simulink model "penduloInvNoLineal"  (Simulink 7.3)
settings: Solver=ode45  StartTime=0.0  StopTime=0.5  RelTol=1e-3
values from neighbouring files (symbols this model uses):
  K = lqr(A,B,Q,R)    [LQR.m]    (also in bestQ.m = setK_lqr(Q_i); graficosPenduloReal.m = setK_lqr(Q_optimo))
libraries: simulink x5
settings Model: Creator=root  LastModifiedBy=Daniel
settings DebuggingCC: FcnCallInpInsideContextMsg=Enable All  StrictBusMsg=ErrorLevel1
settings GRTTargetCC: CombineOutputUpdateFcns=on

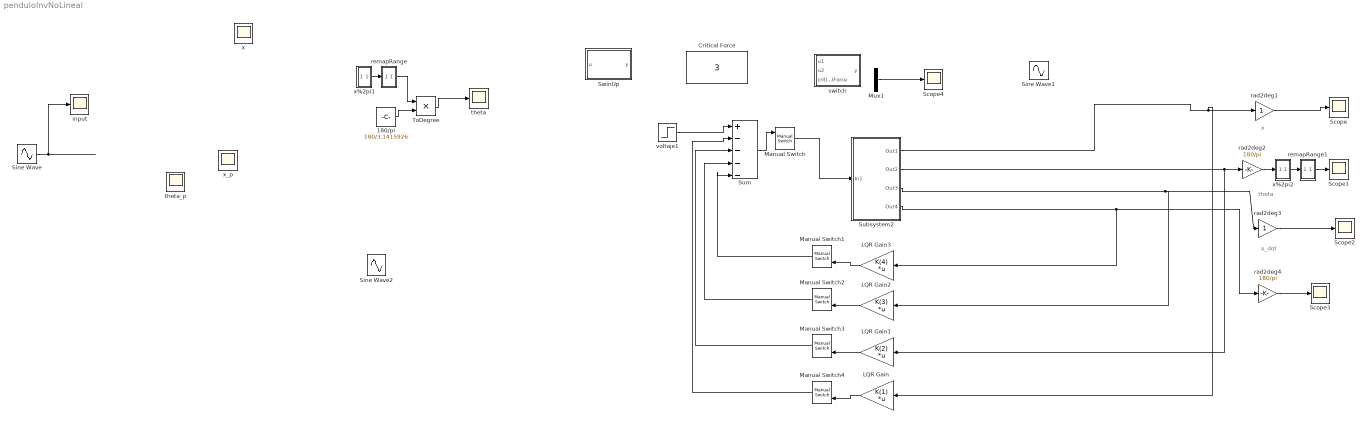
== system penduloInvNoLineal ==
  note: x
  note: theta
  note: x_dot
  180/pi : Constant  Value=180/3.1415926
  Critical Force : Constant  Value=3  OutDataType=fixdt(1, 16)  OutScaling=2^0
  LQR Gain : Gain  Gain=K(1)  Multiplication=Matrix(K*u)  SaturateOnIntegerOverflow=on  OutDataTypeStr=Inherit: Same as input  ParamDataTypeStr=Inherit: Same as input
  LQR Gain1 : Gain  Gain=K(2)  Multiplication=Matrix(K*u)  SaturateOnIntegerOverflow=on  OutDataTypeStr=Inherit: Same as input  ParamDataTypeStr=Inherit: Same as input
  LQR Gain2 : Gain  Gain=K(3)  Multiplication=Matrix(K*u)  SaturateOnIntegerOverflow=on  OutDataTypeStr=Inherit: Same as input  ParamDataTypeStr=Inherit: Same as input
  LQR Gain3 : Gain  Gain=K(4)  Multiplication=Matrix(K*u)  SaturateOnIntegerOverflow=on  OutDataTypeStr=Inherit: Same as input  ParamDataTypeStr=Inherit: Same as input
  Manual Switch : simulink/Signal Routing/Manual Switch  SystemSampleTime=-1  sw=1  action=0  varsize=off
  Manual Switch{1..4} (4 alike) : simulink/Signal Routing/Manual Switch  SystemSampleTime=-1  sw=0  action=0  varsize=off
  Mux1 : Mux  Inputs=2
  Scope{,1..4} (5 alike) : Scope
      Scope settings: SaveName=ScopeData6
      Scope1 settings: SaveName=ScopeData7
      Scope2 settings: SaveName=ScopeData8
      Scope3 settings: SaveName=ScopeData9
      Scope4 settings: SaveName=ScopeData10
  Sine Wave : Sin  Amplitude=0  Bias=0  Frequency=0.25  Phase=0  Samples=10  SampleTime=0.03  Offset=0
  Sine Wave1 : Sin  Amplitude=5  Bias=0  Frequency=1  Phase=0  Samples=10  SampleTime=0  Offset=0
  Sine Wave2 : Sin  Amplitude=2  Bias=0  Frequency=10  Phase=0  Samples=10  SampleTime=0  Offset=0
  Subsystem2 : Subsystem
  Sum : Sum  Inputs=|+----  OutDataType=fixdt(1, 16)  OutScaling=2^0
  SwinUp : Stateflow chart
  ToDegree : Product  RndMeth=Zero
  input : Scope
      settings: SaveName=ScopeData4
  rad2deg1 : Gain  SaturateOnIntegerOverflow=on  OutDataTypeStr=Inherit: Same as input  ParamDataTypeStr=Inherit: Same as input
  rad2deg2 : Gain  Gain=180/pi  SaturateOnIntegerOverflow=on  OutDataTypeStr=Inherit: Same as input  ParamDataTypeStr=Inherit: Same as input
  rad2deg3 : Gain  SaturateOnIntegerOverflow=on  OutDataTypeStr=Inherit: Same as input  ParamDataTypeStr=Inherit: Same as input
  rad2deg4 : Gain  Gain=180/pi  SaturateOnIntegerOverflow=on  OutDataTypeStr=Inherit: Same as input  ParamDataTypeStr=Inherit: Same as input
  remapRange : Stateflow chart  TreatAsAtomicUnit=on
  remapRange1 : Stateflow chart  TreatAsAtomicUnit=on
  switch : Stateflow chart
  theta : Scope
      settings: TimeRange=500  YMin=-200  YMax=200  SaveName=theta
  theta_p : Scope
      settings: SaveName=ScopeData3
  voltaje1 : Step  Time=0  After=1000  SampleTime=0
  x : Scope
  x%2pi1 : Stateflow chart  TreatAsAtomicUnit=on
  x%2pi2 : Stateflow chart  TreatAsAtomicUnit=on
  x_p : Scope
      settings: SaveName=ScopeData2
  wires:
  180/pi/1 -> ToDegree/2
  ToDegree/1 -> theta/1
  x%2pi1/1(y) -> remapRange/1(value)
  remapRange/1(y) -> ToDegree/1
  Sine Wave/1 -> input/1
  ? -> x/1
  ? -> x%2pi1/1(u)
  ? -> x_p/1
  ? -> theta_p/1
  rad2deg4/1 -> Scope3/1
  rad2deg3/1 -> Scope2/1
  Subsystem2/3(Out3) -> LQR Gain2/1, rad2deg3/1
  rad2deg1/1 -> Scope/1
  Mux1/1 -> Scope4/1
  Subsystem2/1(Out1) -> rad2deg1/1, LQR Gain/1
  Subsystem2/2(Out2) -> rad2deg2/1, LQR Gain1/1
  x%2pi2/1(y) -> remapRange1/1(value)
  rad2deg2/1 -> x%2pi2/1(u)
  remapRange1/1(y) -> Scope1/1
  LQR Gain3/1 -> Manual Switch1/2
  LQR Gain2/1 -> Manual Switch2/2
  LQR Gain1/1 -> Manual Switch3/2
  LQR Gain/1 -> Manual Switch4/2
  Manual Switch/1 -> Subsystem2/1(In1)
  Subsystem2/4(Out4) -> rad2deg4/1, LQR Gain3/1
  voltaje1/1 -> Sum/1
  Sum/1 -> Manual Switch/1
  Manual Switch1/1 -> Sum/5
  Manual Switch2/1 -> Sum/4
  Manual Switch3/1 -> Sum/3
  Manual Switch4/1 -> Sum/2

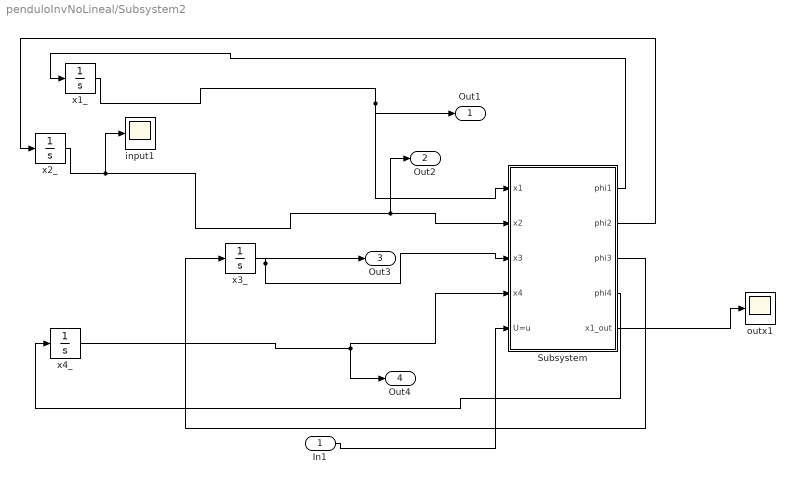
== system penduloInvNoLineal/Subsystem2 ==
  In1 : Inport
  Subsystem : Subsystem
  input1 : Scope
      settings: SaveName=ScopeData5
  outx1 : Scope
  x1_ : Integrator  UpperSaturationLimit=50  LowerSaturationLimit=-50
  x2_ : Integrator  InitialCondition=180.005*pi/180  UpperSaturationLimit=2*pi  LowerSaturationLimit=0
  x3_ : Integrator  UpperSaturationLimit=100  LowerSaturationLimit=-100
  x4_ : Integrator  UpperSaturationLimit=100  LowerSaturationLimit=-100
  Out1 : Outport
  Out2 : Outport  Port=2
  Out3 : Outport  Port=3
  Out4 : Outport  Port=4
  wires:
  x1_/1 -> Subsystem/1(x1), Out1/1
  Subsystem/1(phi1) -> x1_/1
  Subsystem/2(phi2) -> x2_/1
  Subsystem/3(phi3) -> x3_/1
  Subsystem/4(phi4) -> x4_/1
  x4_/1 -> Subsystem/4(x4), Out4/1
  x2_/1 -> input1/1, Subsystem/2(x2), Out2/1
  Subsystem/5(x1_out) -> outx1/1
  In1/1 -> Subsystem/5(U=u)
  x3_/1 -> Out3/1, Subsystem/3(x3)

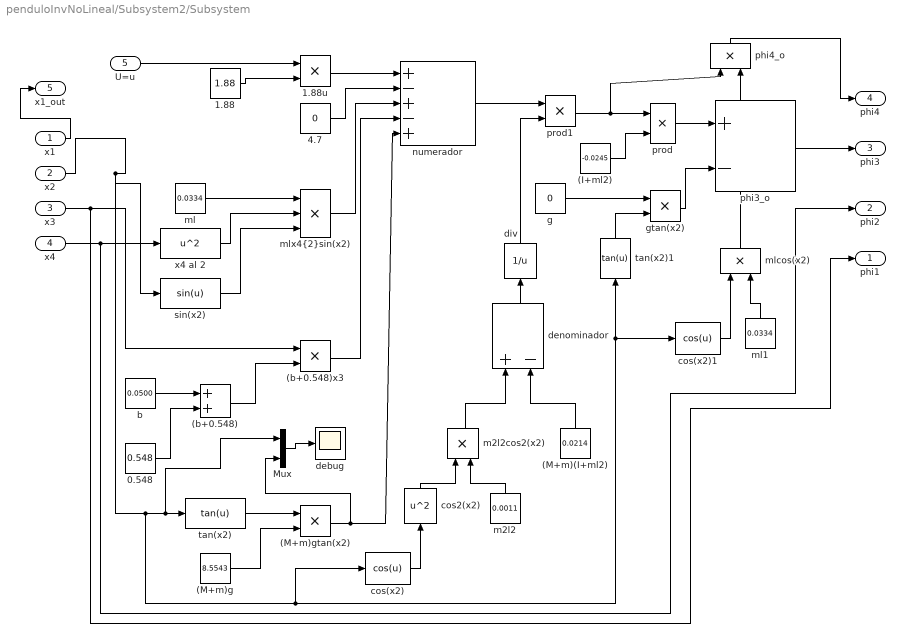
== system penduloInvNoLineal/Subsystem2/Subsystem ==
  x1 : Inport
  x2 : Inport  Port=2
  x3 : Inport  Port=3
  x4 : Inport  Port=4
  U=u : Inport  Port=5
  (I+ml2) : Constant  Value=-0.0245
  (M+m)(I+ml2) : Constant  Value=0.0214
  (M+m)g : Constant  Value=8.5543
  (M+m)gtan(x2) : Product  RndMeth=Zero
  (b+0.548) : Sum
  (b+0.548)x3 : Product  RndMeth=Zero
  0.548 : Constant  Value=0.548
  1.88 : Constant  Value=1.88
  1.88u : Product  RndMeth=Zero
  4.7 : Constant  Value=0
  Mux : Mux  Inputs=2
  b : Constant  Value=0.0500
  cos(x2) : Fcn  Expr=cos(u)  SampleTime=0.1
  cos(x2)1 : Fcn  Expr=cos(u)  SampleTime=0.1
  cos2(x2) : Fcn  Expr=u^2  SampleTime=0.1
  debug : Scope
      settings: SaveName=debug
  denominador : Sum  Inputs=+-
  div : Fcn  Expr=1/u  SampleTime=0.1
  g : Constant  Value=0
  gtan(x2) : Product  RndMeth=Zero
  m2l2 : Constant  Value=0.0011
  m2l2cos2(x2) : Product  RndMeth=Zero
  ml : Constant  Value=0.0334
  ml1 : Constant  Value=0.0334
  mlcos(x2) : Product  RndMeth=Zero
  "mlx4{2}sin(x2)" : Product  Inputs=3  RndMeth=Zero
  numerador : Sum  Inputs=+-+-+
  phi3_o : Sum  Inputs=+-
  phi4_o : Product  RndMeth=Zero
  prod : Product  RndMeth=Zero
  prod1 : Product  RndMeth=Zero
  sin(x2) : Fcn  Expr=sin(u)  SampleTime=0.1
  tan(x2) : Fcn  Expr=tan(u)  SampleTime=0.1
  tan(x2)1 : Fcn  Expr=tan(u)  SampleTime=0.1
  x4 al 2 : Fcn  Expr=u^2  SampleTime=0.1
  phi1 : Outport
  phi2 : Outport  Port=2
  phi3 : Outport  Port=3
  phi4 : Outport  Port=4
  x1_out : Outport  Port=5
  wires:
  1.88/1 -> 1.88u/2
  U=u/1 -> 1.88u/1
  1.88u/1 -> numerador/1
  4.7/1 -> numerador/2
  ml/1 -> "mlx4{2}sin(x2)"/1
  sin(x2)/1 -> "mlx4{2}sin(x2)"/3
  x4 al 2/1 -> "mlx4{2}sin(x2)"/2
  x4/1 -> x4 al 2/1, phi2/1
  "mlx4{2}sin(x2)"/1 -> numerador/3
  (b+0.548)x3/1 -> numerador/4
  x3/1 -> phi1/1, (b+0.548)x3/1
  (b+0.548)/1 -> (b+0.548)x3/2
  b/1 -> (b+0.548)/1
  0.548/1 -> (b+0.548)/2
  (M+m)gtan(x2)/1 -> numerador/5, Mux/2
  tan(x2)/1 -> (M+m)gtan(x2)/1
  (M+m)g/1 -> (M+m)gtan(x2)/2
  (M+m)(I+ml2)/1 -> denominador/2
  m2l2cos2(x2)/1 -> denominador/1
  cos2(x2)/1 -> m2l2cos2(x2)/1
  m2l2/1 -> m2l2cos2(x2)/2
  cos(x2)/1 -> cos2(x2)/1
  numerador/1 -> prod1/1
  prod1/1 -> prod/1, phi4_o/1
  (I+ml2)/1 -> prod/2
  prod/1 -> phi3_o/1
  gtan(x2)/1 -> phi3_o/2
  g/1 -> gtan(x2)/1
  tan(x2)1/1 -> gtan(x2)/2
  mlcos(x2)/1 -> phi4_o/2
  ml1/1 -> mlcos(x2)/2
  cos(x2)1/1 -> mlcos(x2)/1
  phi3_o/1 -> phi3/1
  phi4_o/1 -> phi4/1
  denominador/1 -> div/1
  div/1 -> prod1/2
  x2/1 -> cos(x2)/1, tan(x2)1/1, cos(x2)1/1, tan(x2)/1, Mux/1, sin(x2)/1
  x1/1 -> x1_out/1
  Mux/1 -> debug/1

== matlab function SwinUp ==
  data: u input double; y output double
function y = fcn(u)
%#eml
%y = sin(u);
y=exp(u)*sin(10*u);
end

== matlab function remapRange ==
  data: value input double; y output double
function y = remapRange(value)
    scaleFactor = pi/180;
    if (value>180*scaleFactor)
        %constants
        fromLow = 181*scaleFactor;
        fromHigh = 360*scaleFactor;
        toLow = -179*scaleFactor;
        toHigh = 0*scaleFactor;
        %calculations
        new_range = toHigh-toLow;
        old_range = fromHigh - fromLow;
        new_value = (new_range/old_range)*(value-fromLow)+toLow;
        y = new_value;
    else
        y = value;
    end
        
end

== matlab function x%2pi1 ==
  data: u input double; y output double
function y = fcn(u)
%#codegen

    y = mod(u,2*pi);
end

== matlab function switch ==
  data: u1 input double; y output double; u2 input double; criticalForce input double
function y = fcn(u1,u2,criticalForce)
%#eml

if (abs(u2) < criticalForce) 
    y = u1;
else
    y = u1;
end

== matlab function remapRange1 ==
  data: value input double; y output double
function y = remapRange(value)
    scaleFactor = pi/180;
    if (value>180*scaleFactor)
        %constants
        fromLow = 181*scaleFactor;
        fromHigh = 360*scaleFactor;
        toLow = -179*scaleFactor;
        toHigh = 0*scaleFactor;
        %calculations
        new_range = toHigh-toLow;
        old_range = fromHigh - fromLow;
        new_value = (new_range/old_range)*(value-fromLow)+toLow;
        y = new_value;
    else
        y = value;
    end
        
end

== matlab function x%2pi2 ==
  data: u input double; y output double
function y = fcn(u)
%#codegen

    y = mod(u,2*pi);
end
